simulink model "simPend"  (R2021b)
settings: Solver=VariableStepAuto  StartTime=0.0  StopTime=80.0  RelTol=1e-3
model workspace (MAT data in the model file):
  d = 1
values from neighbouring files (symbols this model uses):
  c = 0.00035    [p1.m]
  g = 9.80665    [p1.m]
  J = 0.0090    (= 0.009)    [p1.m]
  L = 0.495    [p1.m]
  m = 0.43    [p1.m]
libraries: simulink_extras x2, fuzblock x1
settings Model: Creator=mateo  LastModifiedBy=mateo

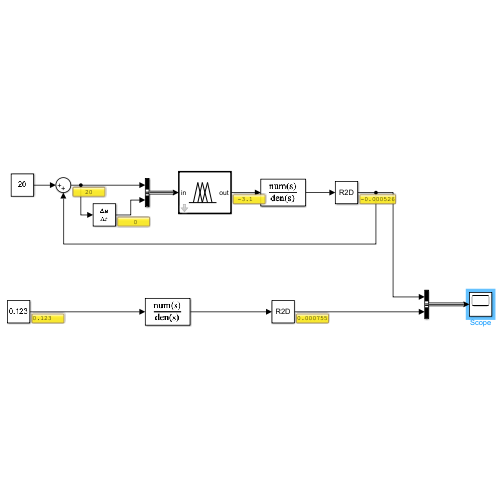
[thumbnail: Simulink's stored preview of the top-level diagram]
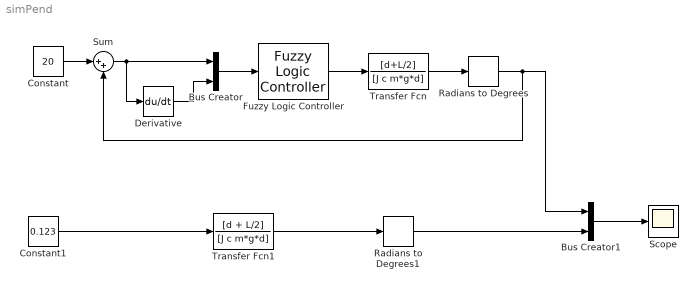
== system simPend ==
  Bus Creator : BusCreator  Inputs=2
  Bus Creator1 : BusCreator  Inputs=2
  Constant : Constant  Value=20
  Constant1 : Constant  Value=0.123  OutMin=[0]  OutMax=[123]
  Derivative : Derivative
  Fuzzy Logic Controller : fuzblock/Fuzzy Logic  Controller  FIS='fuzzy_system.fis'  OutputSampleNumber=101  DataType=double  FuzzifiedInputs=off  RuleFiringStrengths=off  RuleOutputs=off  AggregatedOutputs=off  SimulateUsing=Interpreted execution  OutOfRangeInputValueMessage=warning  NoRuleFiredMessage=warning  EmptyOutputFuzzySetMessage=warning
  Radians to Degrees : simulink_extras/Transformations/Radians to Degrees
  Radians to Degrees1 : simulink_extras/Transformations/Radians to Degrees
  Scope : Scope
  Sum : Sum  Inputs=|++
  Transfer Fcn : TransferFcn  Numerator=[d+L/2]  Denominator=[J c m*g*d]
  Transfer Fcn1 : TransferFcn  Numerator=[d + L/2]  Denominator=[J c m*g*d]
  wires:
  Constant/1 -> Sum/1
  Constant1/1 -> Transfer Fcn1/1
  Sum/1 -> Bus Creator/1, Derivative/1
  Derivative/1 -> Bus Creator/2
  Transfer Fcn/1 -> Radians to Degrees/1
  Radians to Degrees/1 -> Sum/2, Bus Creator1/1
  Transfer Fcn1/1 -> Radians to Degrees1/1
  Radians to Degrees1/1 -> Bus Creator1/2
  Bus Creator1/1 -> Scope/1
  Bus Creator/1 -> Fuzzy Logic Controller/1
  Fuzzy Logic Controller/1 -> Transfer Fcn/1
